simulink model "pick_and_place_Linear_delta_robot"  (R2022b)
settings: Solver=daessc  StartTime=0.0  StopTime=3  FixedStep=dt_solver  RelTol=1e-3  AbsTol=1e-3
model workspace (MAT data in the model file):
  Kd = 0.128272980427
  Ki = 5.87309913441
  Kp = 0.822136815965
  dt_planner = 0.001
  dt_solver = 0.0002
undefined symbols (not defined in the file or in its folder): entire, Marker1, Marker2, Marker3, Marker4, point1, point2, point3, X, Y, Z
libraries: sm_lib x32, nesl_utility x17, Linear_delta_robot_lib x1, slpidlib x1
(part 2 of 2)

== matlab function pick_and_place_Linear_delta_robot/Planning_and_Control/Path Planner ==
  data: eePos input size=3; eePosDes output size=3; eeVelDes output; eeVel input size=3; partPos input size=3; marker1Pos input size=3; marker2Pos input size=3; marker3Pos input size=3; marker4Pos input size=3; t input size=1; eePosGoal output; currentMode output size=1; goalMarker output size=1; suction output size=1
function [eePosDes, eeVelDes, eePosGoal, currentMode, goalMarker, suction] = Planner(eePos, eeVel, partPos, marker1Pos, marker2Pos, marker3Pos, marker4Pos, t)
% Top-level planner.  The end effector goal and suction state depend on
% the current mode: 
%
% mode 0: go to home/initial position (suction off)
% mode 1: go to part (suction off)
% mode 2: move part to goal position (suction on)
%
% When a mode is first entered, a new end effector trajectory is planned.
% This is done by first computing a 3rd order polynomial curve c(s)
% corresponding to the desired path (in xyz camera coordinates) of the end
% effector from its current position to the goal position for that mode.
% Then a 5th order polynomial s(t) is computed which serves as the
% time-scaling along the path.  The time-scaling is computed such that the
% initial and final velocities and accelerations along the path are zero.
% This results in the desired trajectory c(s(t)) = c(t).  For a given time,
% this function returns the corresponding position (c(t) = eePosDes) and
% velocity (c'(t) = eeVelDes) of the trajectory.

% Copyright 2020-2021 The MathWorks, Inc.

persistent mode plan homePos pickAndDropZGoal ...
    marker1PosGoal marker2PosGoal marker3PosGoal marker4PosGoal ...
    marker5PosGoal nextMarker stayHome

if isempty(mode)
    mode = 0;
    plan = true;
    pickAndDropZGoal = partPos(3) - 0.001;
    marker4PosGoal = [marker1Pos(1:2); pickAndDropZGoal];
    marker3PosGoal = [marker2Pos(1:2); pickAndDropZGoal];
    marker2PosGoal = [marker3Pos(1:2); pickAndDropZGoal];
    marker1PosGoal = [marker4Pos(1:2); pickAndDropZGoal];
    marker5PosGoal = [partPos(1:2); pickAndDropZGoal];
    homePos = eePos;
    nextMarker = 0;
    stayHome = false;
end

switch mode
    case 0
        % Go to home position
        suction = 0;
        eePosGoal = homePos;
        startVertical = false;
        endVertical = false;
        [eePosDes, eeVelDes, done] = gotoPosition(eePosGoal, eePos, eeVel, t, startVertical, endVertical, plan);
        plan = false;
        if done
            if ~stayHome
                mode = 1;
                plan = true;
            end
        end
        
    case 1
        % Move to just above part and hover (end of path is vertical)
        eePosGoal = [partPos(1:2); pickAndDropZGoal];
        suction = 0;
        startVertical = false;
        endVertical = true;
        [eePosDes, eeVelDes, done] = gotoPosition(eePosGoal, eePos, eeVel, t, startVertical, endVertical, plan);
        plan = false;
        if done
            nextMarker = 1;
            mode = 2;
            plan = true;
        end
        
    case 2
        % Grasp part and move it to the next marker (beginning and end of
        % path are vertical)
        switch nextMarker
            case 1
                eePosGoal = marker1PosGoal;
            case 2
                eePosGoal = marker2PosGoal;
            case 3
                eePosGoal = marker3PosGoal;
            case 4
                eePosGoal = marker4PosGoal;
            case 6
                eePosGoal = marker5PosGoal;
            otherwise
                error('invalid nextMarker')
        end
        suction = 1;
        startVertical = true;
        endVertical = true;
        [eePosDes, eeVelDes, done] = gotoPosition(eePosGoal, eePos, eeVel, t, startVertical, endVertical, plan);
        plan = false;
        if done
            nextMarker = nextMarker + 1;
            if nextMarker == 5
                nextMarker = 6;
                stayHome = true;
            end
            if nextMarker == 7 && stayHome
                nextMarker = 0;
                mode = 0;
            end
            plan = true;
        end
        
    otherwise
        error('invalid mode')
end

currentMode = mode;
goalMarker = nextMarker;
end


function p = getPoly5(t0,tf,x0,v0,a0,xf,vf,af)
% Compute the 5th order polynomial 
% 
% poly(t) = a*t^5 + b*t^4 + c*t^3 + d*t^2 + e*t + f
%
% such that
%
% p(t0) = x0; p(tf) = xf
% p'(t0) = v0; p'(tf) = vf
% p''(to) = a0; p''(tf) = af
%
% Returns the coeffecient vector p = [a b c d e f]

A = [t0^5    t0^4    t0^3   t0^2 t0 1;
     5*t0^4  4*t0^3  3*t0^2 2*t0 1  0;
     20*t0^3 12*t0^2 6*t0   2    0  0;
     tf^5    tf^4    tf^3   tf^2 tf 1;
     5*tf^4  4*tf^3  3*tf^2 2*tf 1  0;
     20*tf^3 12*tf^2 6*tf   2    0  0];
b = [x0 v0 a0 xf vf af]';
p = A\b;
end

function p = getPoly3(t0,tf,x0,v0,xf,vf)
% Compute the 3rd order polynomial 
% 
% poly(t) = a*t^3 + b*t^2 + c*t + d
%
% such that
%
% p(t0) = x0; p(tf) = xf
% p'(t0) = v0; p'(tf) = vf
%
% Returns the coeffecient vector p = [a b c d]

A = [t0^3   t0^2 t0 1;
     3*t0^2 2*t0 1  0;
     tf^3   tf^2 tf 1;
     3*tf^2 2*tf 1  0];
b = [x0 v0 xf vf]';
p = A\b;
end

function [eePosDes, eeVelDes, atGoal] = gotoGoal(...
    plan, ...
    t, timeToGoal, ...
    eePos, eeVel, ...
    eePosGoal, startDirectionGoal, endDirectionGoal)
% Return desired position and velocity at the current time along the
% trajectory to a goal position.  The trajectory is only computed if 'plan'
% is true.  The trajectory is determined by the desired time to reach the
% goal (timeToGoal), the desired goal position (eePosGoal), and the
% starting and ending directions (startDirectionGoal and endDirectionGoal)
% of the curve to the goal in xyz camera coordinates.  It always assumed
% that the initial and final velocities and accelerations along the
% trajectory are zero.  Thus, the goal velocity is always zero.  If the
% current position and velocity are sufficiently close to the goal position
% and velocity, 'atGoal' is true.

persistent cpoly cdpoly spoly sdpoly t0 tf maxErrPos maxErrVel

if isempty(tf)
    cpoly = zeros(3,4);
    cdpoly = zeros(3,3);
    spoly = zeros(1,6);
    sdpoly = zeros(1,5);
    
    t0 = t;
    tf = t;
    
    maxErrPos = 0.002;
    maxErrVel = 0.01;
end

errPos = eePosGoal - eePos;
errVel = -eeVel;
errPosNorm = norm(errPos);
errVelNorm = norm(errVel);

if plan
    t0 = t;
    tf = t0 + timeToGoal;
    [cpoly, cdpoly, spoly, sdpoly] = getTrajectory(...
        t0, tf, eePos, eePosGoal, startDirectionGoal, endDirectionGoal);
end

t = min(t,tf); %if t > tf, we just want to keep aiming for end of trajectory
s = polyval(spoly,t);
eePosDes = [polyval(cpoly(1,:),s);polyval(cpoly(2,:),s);polyval(cpoly(3,:),s)];
eeVelDes = [polyval(cdpoly(1,:),s);polyval(cdpoly(2,:),s);polyval(cdpoly(3,:),s)]*polyval(sdpoly,t);
atGoal = errPosNorm < maxErrPos && errVelNorm < maxErrVel;
end

function [cpoly, cdpoly, spoly, sdpoly] = getTrajectory(...
    t0, tf, eePos, eePosGoal, startDirectionGoal, endDirectionGoal)
% Return polynomials needed to compute a time-scaled trajectory
% from eePos to eePosGoal such that initial and final velocities
% and accelerations are zero.  The path of the trajectory in xyz space has
% an initial tangent equal to startDirectionGoal and an ending tangent of
% endDirectionGoal.
%
% Let c(s) = [x(s);y(s);z(s)] with s = [0 1] be a curve in xyz space from
% eePos to eePosGoal.  We assume each element is a 3rd order
% polymonial and compute the corresponding 3-by-4 coefficient matrix,
% cpoly:
%
%         [a1*s^3 + b1*s^2 + c1*s + d1]           [s^3]
%  c(s) = [a2*s^3 + b2*s^2 + c2*s + d2] = cpoly * [s^2]
%         [a3*s^3 + b3*s^2 + c3*s + d3]           [s  ]
%                                                 [1  ]
%
% The 12 coefficeints in cpoly are uniquely determined by the following
% boundary conditions:
%
% c(0) = eePos
% c(1) = eePosGoal
% c'(0) = startDirectionGoal
% c'(1) = endDirectionGoal
%
% cdpoly is a 3-by-3 matrix of polynomial coefficents of the derivatives of
% each row of cpoly:
%
%          [3*a1 2*b1 c1]
% cdpoly = [3*a2 2*b2 c2]
%          [3*a3 2*b3 c3]
%
% The curve c(s) is then time-scaled to ensure that the initial and final
% speeds and accelerations along the curve are zero.  The time scaling
% s(t) is a 5th order polynomial
%
%  s(t) = A*s^5 + B*s^4 + C*s^3 + D*s^2 + E*s + F
%
%       = spoly*[s^5 s^4 s^3 s^2 s 1]'
%
% spoly is a 1-by-6 vector of coefficents with values uniquely determined
% by the following boundary conditions:
%
% s(t0) = 0
% s(tf) = 1
% s'(t0) = 0
% s'(tf) = 0
% s''(t0) = 0
% s''(tf) = 0
%
% sdpoly is a 1-by-5 matrix of polynomial coefficents of the derivative of
% spoly:
%
% sdpoly = [5*A 4*B 3*C 2*D E]
%
% The final time-scaled trajectory corresponds to c(s(t))

s0 = 0;
sf = 1;
c0 = eePos;
cf = eePosGoal;
cd0 = startDirectionGoal;
cdf = endDirectionGoal;
cpoly = zeros(3,4);
cdpoly = zeros(3,3);
for i = 1:3
    cpoly(i,:) = getPoly3(s0,sf,c0(i),cd0(i),cf(i),cdf(i));
    % Need to be careful with polyder.  If the polynomial is equivalent
    % to just a constant (e.g., [0 0 0 1]), then polyder returns [0]
    % instead of [0 0 0].
    pd = polyder(cpoly(i,:));
    if length(pd) == 3
        cdpoly(i,:) = pd;
    else
        cdpoly(i,:) = [0 0 0];
    end
end

s0 = 0;
sf = 1;
sd0 = 0;
sdf = 0;
sdd0 = 0;
sddf = 0;
spoly = getPoly5(t0,tf,s0,sd0,sdd0,sf,sdf,sddf);
sdpoly = polyder(spoly);
end

function [eePosDes, eeVelDes, done] = gotoPosition(eePosGoal, eePos, eeVel, t, startVertical, endVertical, plan)
% High-level function to go to a goal position.  Returns the desired
% position and velocity at the current time along the trajectory to a goal
% position. The time to goal along the trajectory is always set to 0.2
% seconds.  The trajectory to the goal is replanned whenever plan is true.
% startVertical and endVertical indicate whether the curve defined by the
% trajectory should begin and/or end vertically (i.e., the end effector
% should move straight up or down when starting or ending its motion).  It
% is always assumed that the initial and final velocities and accelerations
% along the trajectory are zero.  Thus, the goal velocity is always zero.
% If the current position and velocity are sufficiently close to the goal
% position and velocity, 'done' is true.

if startVertical
    startDirectionGoal = [0;0;-0.2];
else
    startDirectionGoal = eeVel;
end
if endVertical
    endDirectionGoal = [0;0;0.2];
else
    endDirectionGoal = [0;0;0];
end
timeToGoal = 0.2;
[eePosDes, eeVelDes, atGoal] = gotoGoal(...
    plan, ...
    t, timeToGoal, ...
    eePos, eeVel, ...
    eePosGoal, startDirectionGoal, endDirectionGoal);
done = atGoal;
end

== matlab function pick_and_place_Linear_delta_robot/Planning_and_Control/Forward Kinematics ==
  data: actuatorPos input size=3; eePos output size=3; actuatorVel input size=3; eeVel output
function [eePos, eeVel] = FK(actuatorPos, actuatorVel)
% Wrapper around sm_pick_and_place_fk.m, which creates a persistent
% KinematicsSolver object for the forwards kinematics problem and then
% solves it.

coder.extrinsic('analytic_linear_delta_robot_fk');
persistent init
if isempty(init)
    init = true;
    eePos = zeros(3,1);
    eeVel = zeros(3,1);
    status = 1;
end
[eePos, eeVel, status] = analytic_linear_delta_robot_fk(actuatorPos, actuatorVel);
if status ~= 1
    error('fk solve failed')
end

== matlab function pick_and_place_Linear_delta_robot/Planning_and_Control/Inverse Kinematics ==
  data: eePosDes input size=3; actuatorPosDes output size=3
function actuatorPosDes  = IK(eePosDes)
% Wrapper around sm_pick_and_place_ik.m, which creates a persistent
% KinematicsSolver object for the inverse kinematics problem and then
% solves it.

coder.extrinsic('analytic_linear_delta_robot_ik');
persistent init
if isempty(init)
    init = true;
    actuatorPosDes = zeros(3,1);
    guessValsOut = zeros(3,1);
    status = 1;
end
[actuatorPosDes, status] = analytic_linear_delta_robot_ik(eePosDes);
if status ~= 1
    error('ik solve failed');
end
